simulink model "q_as_ol"  (Simulink 7.8)
settings: Solver=ode1  StartTime=0.0  StopTime=30  FixedStep=0.001  RelTol=1e-3
undefined symbols (not defined in the file): A, B, C, D, HIL, qc_get_step_size
libraries: simulink x11, quarc_library x9
settings Model: Creator=DCrymble  LastModifiedBy=pmartin  SimulationMode=external  ExtModeTrigDuration=50000  BufferReuse=off
settings SolverCC: PositivePriorityOrder=on
settings OptimizationCC: BooleanDataType=off  InlineInvariantSignals=on  OptimizeBlockIOStorage=off  BufferReuse=off  ExpressionFolding=off  LocalBlockOutputs=off  InitFltsAndDblsToZero=on
settings DebuggingCC: FcnCallInpInsideContextMsg=Use local settings  StrictBusMsg=Warning
settings SFSimCC: SimParseCustomCode=off
settings RTWCC: SystemTargetFile=quarc_windows.tlc  TemplateMakefile=quarc_default_tmf  Description=QuaRC Win32 Target  ProcessScript=quarc_windows_make_rtw_hook
settings STFCustomTargetCC: TargetPreCompLibLocation=C:\PROGRA~2\QUARC\lib\2012b\windows\release  SystemTargetFile=quarc_windows.tlc
settings GRTTargetCC: TargetPreCompLibLocation=C:\PROGRA~2\QUARC\lib\2012b\windows\release  ParMdlRefBuildCompliant=off  CompOptLevelCompliant=off  ConcurrentExecutionCompliant=off  MatFileLogging=off  ExtMode=on  ExtModeMexFile=quarc_comm

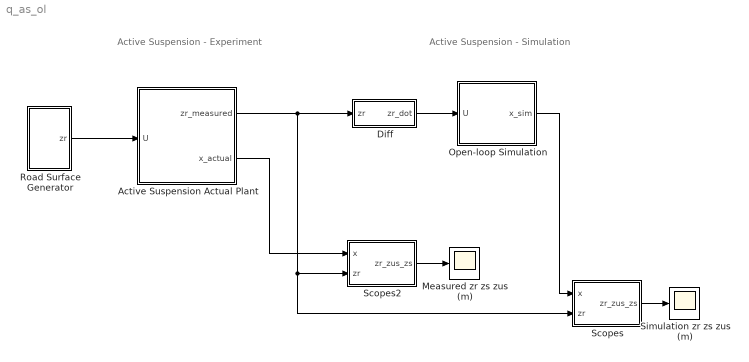
== system q_as_ol ==
  note: Active Suspension - Experiment
  note: Active Suspension - Simulation
  Active Suspension Actual Plant : Subsystem
  Diff : Subsystem
  Measured zr zs zus (m) : Scope
      settings: YMin=-0.0225  YMax=0.0325  SaveName=ScopeData3  MaxDataPoints=300000
  Open-loop Simulation : Subsystem
  Road Surface Generator : Subsystem
  Scopes : Subsystem
  Scopes2 : Subsystem
  Simulation zr zs zus (m) : Scope
      settings: YMin=-0.0225  YMax=0.0325  SaveName=ScopeData4  MaxDataPoints=300000
  wires:
  Open-loop Simulation/1(x_sim) -> Scopes/1(x)
  Active Suspension Actual Plant/1(zr_measured) -> Scopes/2(zr), Scopes2/2(zr), Diff/1(zr)
  Active Suspension Actual Plant/2(x_actual) -> Scopes2/1(x)
  Scopes2/1(zr_zus_zs) -> Measured zr zs zus (m)/1
  Scopes/1(zr_zus_zs) -> Simulation zr zs zus (m)/1
  Road Surface Generator/1(zr) -> Active Suspension Actual Plant/1(U)
  Diff/1(zr_dot) -> Open-loop Simulation/1(U)

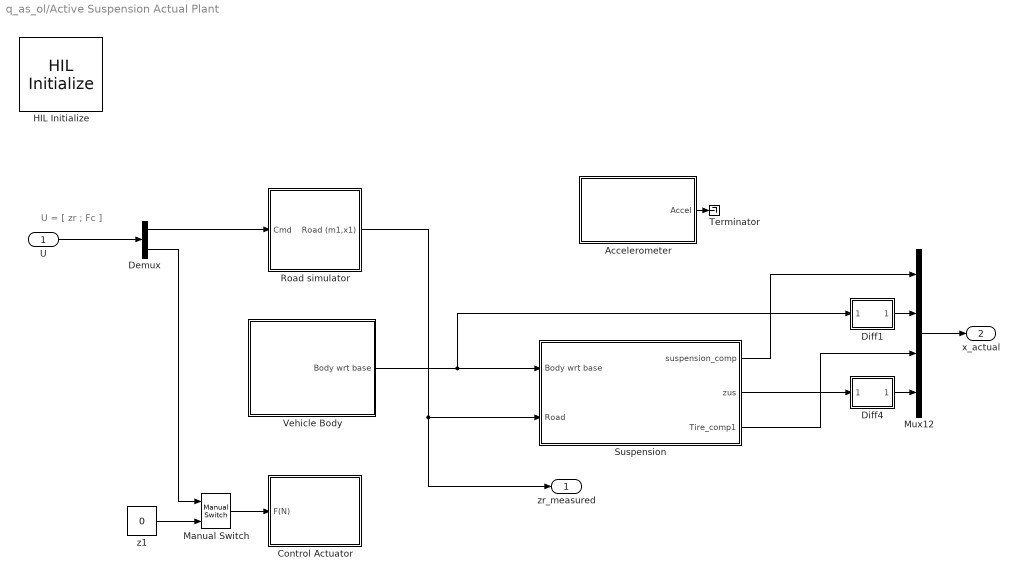
== system q_as_ol/Active Suspension Actual Plant ==
  note: U = [ zr ; Fc ]
  U : Inport
  Accelerometer : Subsystem
  Control Actuator : Subsystem
  Demux : Demux  Outputs=2
  Diff1 : Subsystem
  Diff4 : Subsystem
  HIL Initialize : quarc_library/Data Acquisition/Generic/Configuration/HIL Initialize  Priority=-99  object_name=HIL-1  board_type=q8_usb  board_number=0  board_options=update_rate=normal;decimation=1  exclusive=off  active=off  hardware_clocks=[0:2]  clock_modes=[]  initial_clock_frequencies=[]  set_clock_params_at_start=off  set_clock_params_at_switch_in=off  set_clock_frequencies_at_start=off  set_clock_frequencies_at_switch_in=off  analog_input_channels=[0:7]  analog_input_maximums=10  analog_input_minimums=-10  set_analog_input_params_at_start=on  set_analog_input_params_at_switch_in=off  analog_output_channels=[0:7]  analog_output_maximums=10  analog_output_minimums=-10  initial_analog_outputs=[0]  final_analog_outputs=[0]  watchdog_analog_outputs=0  set_analog_output_params_at_start=on  set_analog_output_params_at_switch_in=off  set_analog_outputs_at_start=on  set_analog_outputs_at_switch_in=off  set_analog_outputs_at_terminate=on  set_analog_outputs_at_switch_out=off  set_analog_outputs_on_watchdog=off  digital_input_channels=[]  digital_output_channels=[0:4]  digital_output_configuration=[]  initial_digital_outputs=[0 0 0 0 1]  final_digital_outputs=[1 1 1 1 0]  watchdog_digital_outputs=[1 1 1 1 0]  set_digital_output_params_at_start=off  set_digital_output_params_at_switch_in=off  set_digital_outputs_at_start=on  set_digital_outputs_at_switch_in=off  set_digital_outputs_at_terminate=on  set_digital_outputs_at_switch_out=off  set_digital_outputs_on_watchdog=off  encoder_channels=[0:7]  quadrature=[4]  encoder_filter_frequency=[]  initial_encoder_counts=[0]  set_encoder_params_at_start=on  set_encoder_params_at_switch_in=off  set_encoder_counts_at_start=on  set_encoder_counts_at_switch_in=off  pwm_channels=[0:7]  pwm_modes=0  pwm_frequency=99.532799999999995e6/4095  pwm_configuration=[0]  pwm_alignment=[0]  pwm_polarity=[1]  pwm_leading_deadband=[0]  pwm_trailing_deadband=[0]  initial_pwm_outputs=[0]  final_pwm_outputs=[0]  watchdog_pwm_outputs=[0]  set_pwm_params_at_start=on  set_pwm_params_at_switch_in=off  set_pwm_outputs_at_start=on  set_pwm_outputs_at_switch_in=off  set_pwm_outputs_at_terminate=on  set_pwm_outputs_at_switch_out=off  set_pwm_outputs_on_watchdog=off  other_output_channels=[]  initial_other_outputs=[]  final_other_outputs=[]  watchdog_other_outputs=[]  set_other_outputs_at_start=off  set_other_outputs_at_switch_in=off  set_other_outputs_at_terminate=off  set_other_outputs_at_switch_out=off  set_other_outputs_on_watchdog=off
  Manual Switch : simulink/Signal Routing/Manual Switch  sw=1  action=0  varsize=off
  Mux12 : Mux
  Road simulator : Subsystem
  Suspension : Subsystem
  Terminator : Terminator
  Vehicle Body : Subsystem
  z1 : Constant  Value=0
  zr_measured : Outport
  x_actual : Outport  Port=2
  wires:
  Manual Switch/1 -> Control Actuator/1(F(N))
  z1/1 -> Manual Switch/2
  Suspension/1(suspension_comp) -> Mux12/1
  Vehicle Body/1(Body wrt base) -> Diff1/1(In1), Suspension/1("Body wrt base ")
  Diff1/1(Out2) -> Mux12/2
  Diff4/1(Out2) -> Mux12/4
  Suspension/2(zus) -> Diff4/1(In1)
  Mux12/1 -> x_actual/1
  Suspension/3(Tire_comp1) -> Mux12/3
  U/1 -> Demux/1
  Road simulator/1(Road (m1,x1)) -> zr_measured/1, Suspension/2(Road)
  Accelerometer/1(Accel) -> Terminator/1
  Demux/1 -> Road simulator/1(Cmd)
  Demux/2 -> Manual Switch/1

== system q_as_ol/Diff ==
  zr : Inport
  2nd Order Filter Input ICs3 : Subsystem
  Constant : Constant  Value=0
  Constant3 : Constant  Value=1000
  Mux : Mux  Inputs=2
  Terminator_1 : Terminator
  z4 : Constant
  zr_dot : Outport
  wires:
  Constant3/1 -> 2nd Order Filter Input ICs3/2(Wn)
  z4/1 -> 2nd Order Filter Input ICs3/3(z)
  zr/1 -> 2nd Order Filter Input ICs3/1(In)
  2nd Order Filter Input ICs3/1(Out) -> Terminator_1/1
  Mux/1 -> zr_dot/1
  2nd Order Filter Input ICs3/2(Out_dot) -> Mux/1
  Constant/1 -> Mux/2

== system q_as_ol/Open-loop Simulation ==
  U : Inport
  Demux : Demux  Outputs=[4 2]
  Open-Loop  State-Space : StateSpace  A=A  B=B  C=cat(1,eye(4), C)  D=D
  Terminator : Terminator
  Unit Delay : UnitDelay  SampleTime=-1
  x_sim : Outport
  wires:
  Open-Loop  State-Space/1 -> Demux/1
  Demux/1 -> Unit Delay/1
  U/1 -> Open-Loop  State-Space/1
  Unit Delay/1 -> x_sim/1
  Demux/2 -> Terminator/1

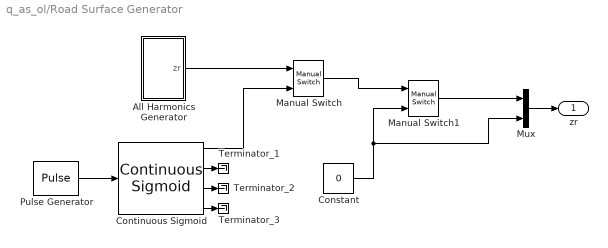
== system q_as_ol/Road Surface Generator ==
  All Harmonics Generator : Subsystem
  Constant : Constant  Value=0
  Continuous Sigmoid : quarc_library/Sources/Sigmoids/Continuous Sigmoid  params_source=Internal (dialog parameters)  max_velocity=.6/3  max_acceleration=20  initial_position=0  initial_velocity=0  hold_off=0.5  input_sample_time=-1  output_sample_time=qc_get_step_size
  Manual Switch : simulink/Signal Routing/Manual Switch  sw=1  action=0  varsize=off
  Manual Switch1 : simulink/Signal Routing/Manual Switch  sw=1  action=0  varsize=off
  Mux : Mux  Inputs=2
  Pulse Generator : DiscretePulseGenerator  PulseType=Time based  Amplitude=0.02  Period=3  PulseWidth=50  PhaseDelay=.1
  Terminator_1 : Terminator
  Terminator_2 : Terminator
  Terminator_3 : Terminator
  zr : Outport
  wires:
  Pulse Generator/1 -> Continuous Sigmoid/1
  All Harmonics Generator/1(zr) -> Manual Switch/1
  Continuous Sigmoid/1 -> Manual Switch/2
  Constant/1 -> Mux/2, Manual Switch1/2
  Manual Switch/1 -> Manual Switch1/1
  Continuous Sigmoid/2 -> Terminator_1/1
  Continuous Sigmoid/3 -> Terminator_2/1
  Continuous Sigmoid/4 -> Terminator_3/1
  Mux/1 -> zr/1
  Manual Switch1/1 -> Mux/1

== system q_as_ol/Scopes ==
  x : Inport
  zr : Inport  Port=2
  Demux : Demux
  Mux1 : Mux  Inputs=3
  Sum1 : Sum  Inputs=2  SaturateOnIntegerOverflow=on  InputSameDT=on  OutDataTypeStr=Inherit: Same as first input
  Sum3 : Sum  Inputs=3  SaturateOnIntegerOverflow=on  InputSameDT=on  OutDataTypeStr=Inherit: Same as first input
  Terminator : Terminator
  Terminator1 : Terminator
  zr_zus_zs : Outport
  wires:
  Demux/1 -> Sum3/2
  Demux/3 -> Sum3/3, Sum1/2
  zr/1 -> Mux1/1, Sum3/1, Sum1/1
  x/1 -> Demux/1
  Sum1/1 -> Mux1/2
  Sum3/1 -> Mux1/3
  Mux1/1 -> zr_zus_zs/1
  Demux/2 -> Terminator/1
  Demux/4 -> Terminator1/1

== system q_as_ol/Scopes2 ==
  x : Inport
  zr : Inport  Port=2
  Demux : Demux
  Mux1 : Mux  Inputs=3
  Sum1 : Sum  Inputs=2  SaturateOnIntegerOverflow=on  InputSameDT=on  OutDataTypeStr=Inherit: Same as first input
  Sum3 : Sum  Inputs=3  SaturateOnIntegerOverflow=on  InputSameDT=on  OutDataTypeStr=Inherit: Same as first input
  Terminator : Terminator
  Terminator1 : Terminator
  zr_zus_zs : Outport
  wires:
  Mux1/1 -> zr_zus_zs/1
  Sum3/1 -> Mux1/3
  Sum1/1 -> Mux1/2
  x/1 -> Demux/1
  zr/1 -> Sum1/1, Sum3/1, Mux1/1
  Demux/3 -> Sum1/2, Sum3/3
  Demux/1 -> Sum3/2
  Demux/2 -> Terminator/1
  Demux/4 -> Terminator1/1

== system q_as_ol/Active Suspension Actual Plant/Accelerometer ==
  Bias Removal : quarc_library/Discrete/Bias Removal  start_time=0  end_time=.099  switch_id=0  sample_time=qc_get_step_size
  HIL Read Analog : quarc_library/Data Acquisition/Generic/Immediate I//O/HIL Read Analog  object_name=HIL-1  channels=0  sample_time=qc_get_step_size  active=on  vector_output=off
  Terminator : Terminator
  Terminator1 : Terminator
  filter : Subsystem
  mm/sec1 : Gain  Gain=-9.8
  Accel : Outport
  wires:
  Bias Removal/1 -> filter/1(In1)
  filter/1(Out2) -> mm/sec1/1
  mm/sec1/1 -> Accel/1
  HIL Read Analog/1 -> Bias Removal/1
  Bias Removal/2 -> Terminator/1
  Bias Removal/3 -> Terminator1/1

== system q_as_ol/Active Suspension Actual Plant/Control Actuator ==
  F(N) : Inport
  A/V : Gain  Gain=-2
  A/V1 : Gain  Gain=1/19.16
  Amp : Scope
      settings: TimeRange=5  YMin=-1  YMax=1.25  SaveName=ScopeData9
  Force : Scope
      settings: TimeRange=5  YMin=-15  YMax=15  SaveName=ScopeData5
  HIL Write Analog1 : quarc_library/Data Acquisition/Generic/Immediate I//O/HIL Write Analog  object_name=HIL-1  channels=0  sample_time=-1  active=off  vector_input=on
  Saturation2 : Saturate  UpperLimit=5  LowerLimit=-5
  wires:
  Saturation2/1 -> Amp/1, A/V/1
  A/V1/1 -> Saturation2/1
  F(N)/1 -> Force/1, A/V1/1
  A/V/1 -> HIL Write Analog1/1

== system q_as_ol/Active Suspension Actual Plant/Diff1 ==
  In1 : Inport
  2nd Order Filter Input ICs3 : Subsystem
  Constant3 : Constant  Value=500
  Terminator_1 : Terminator
  z4 : Constant
  Out2 : Outport
  wires:
  2nd Order Filter Input ICs3/2(Out_dot) -> Out2/1
  In1/1 -> 2nd Order Filter Input ICs3/1(In)
  z4/1 -> 2nd Order Filter Input ICs3/3(z)
  Constant3/1 -> 2nd Order Filter Input ICs3/2(Wn)
  2nd Order Filter Input ICs3/1(Out) -> Terminator_1/1

== system q_as_ol/Active Suspension Actual Plant/Diff4 ==
  In1 : Inport
  2nd Order Filter Input ICs3 : Subsystem
  Constant3 : Constant  Value=500
  Terminator_1 : Terminator
  z4 : Constant
  Out2 : Outport
  wires:
  Constant3/1 -> 2nd Order Filter Input ICs3/2(Wn)
  z4/1 -> 2nd Order Filter Input ICs3/3(z)
  In1/1 -> 2nd Order Filter Input ICs3/1(In)
  2nd Order Filter Input ICs3/2(Out_dot) -> Out2/1
  2nd Order Filter Input ICs3/1(Out) -> Terminator_1/1

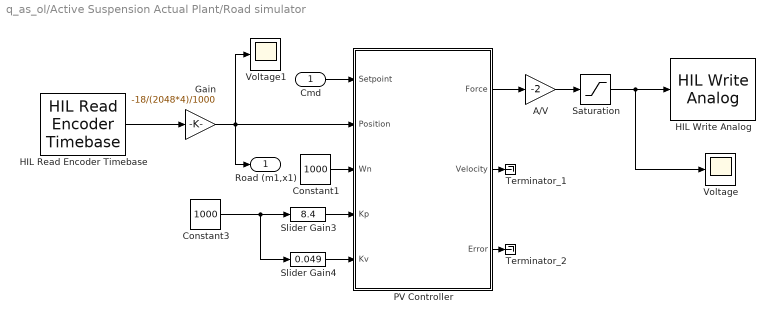
== system q_as_ol/Active Suspension Actual Plant/Road simulator ==
  Cmd : Inport
  A/V : Gain  Gain=-2
  Constant1 : Constant  Value=1000
  Constant3 : Constant  Value=1000
  Gain : Gain  Gain=-18/(2048*4)/1000
  HIL Read Encoder Timebase : quarc_library/Data Acquisition/Generic/Timebases/HIL Read Encoder Timebase  object_name=HIL-1  clock=[0]  channels=1  samples_in_buffer=max(ceil(1/qc_get_step_size), 1)  active=on  vector_output=on  data_type_mode=Inherit via back propagation  data_type=double
  HIL Write Analog : quarc_library/Data Acquisition/Generic/Immediate I//O/HIL Write Analog  object_name=HIL-1  channels=1  sample_time=-1  active=off  vector_input=on
  PV Controller : Subsystem
  Saturation : Saturate  UpperLimit=10  LowerLimit=-10
  Slider Gain3 : simulink/Math Operations/Slider Gain  low=0  gain=8.4  high=70
  Slider Gain4 : simulink/Math Operations/Slider Gain  low=0  gain=0.049  high=0.1
  Terminator_1 : Terminator
  Terminator_2 : Terminator
  Voltage : Scope
      settings: TimeRange=1  YMin=-10  YMax=-10
  Voltage1 : Scope
      settings: TimeRange=5  YMin=-0.0005  YMax=0.0105  SaveName=ScopeData16  MaxDataPoints=50000
  Road (m1,x1) : Outport
  wires:
  A/V/1 -> Saturation/1
  Constant1/1 -> PV Controller/3(Wn)
  Gain/1 -> PV Controller/2(Position), Road (m1,x1)/1, Voltage1/1
  Slider Gain3/1 -> PV Controller/4(Kp)
  Constant3/1 -> Slider Gain4/1, Slider Gain3/1
  Slider Gain4/1 -> PV Controller/5(Kv)
  HIL Read Encoder Timebase/1 -> Gain/1
  Saturation/1 -> HIL Write Analog/1, Voltage/1
  Cmd/1 -> PV Controller/1(Setpoint)
  PV Controller/1(Force) -> A/V/1
  PV Controller/2(Velocity) -> Terminator_1/1
  PV Controller/3(Error) -> Terminator_2/1

== system q_as_ol/Active Suspension Actual Plant/Suspension ==
  "Body wrt base " : Inport
  Road : Inport  Port=2
  HIL Read Encoder : quarc_library/Data Acquisition/Generic/Immediate I//O/HIL Read Encoder  object_name=HIL-1  channels=0  sample_time=qc_get_step_size  active=on  vector_output=off  data_type_mode=Inherit via back propagation  data_type=double
  Sum : Sum  Inputs=|+-
  Sum1 : Sum  Inputs=|+-
  count2m : Gain  Gain=12*pi/4000/1000
  susp_comp : Scope
      settings: YMin=-0.02  YMax=0.0125  SaveName=ScopeData11
  suspension_comp : Outport
  zus : Outport  Port=2
  Tire_comp1 : Outport  Port=3
  wires:
  Sum/1 -> zus/1, Sum1/1
  "Body wrt base "/1 -> Sum/1
  HIL Read Encoder/1 -> count2m/1
  count2m/1 -> Sum/2, suspension_comp/1, susp_comp/1
  Road/1 -> Sum1/2
  Sum1/1 -> Tire_comp1/1

== system q_as_ol/Active Suspension Actual Plant/Vehicle Body ==
  Body wrt base1 : Scope
      settings: YMin=-0.006  YMax=0.017  SaveName=ScopeData8
  HIL Read Encoder : quarc_library/Data Acquisition/Generic/Immediate I//O/HIL Read Encoder  object_name=HIL-1  channels=2  sample_time=qc_get_step_size  active=on  vector_output=off  data_type_mode=Inherit via back propagation  data_type=double
  count2m : Gain  Gain=pi()*25.4/4/4096/1000
  Body wrt base : Outport
  wires:
  HIL Read Encoder/1 -> count2m/1
  count2m/1 -> Body wrt base/1, Body wrt base1/1

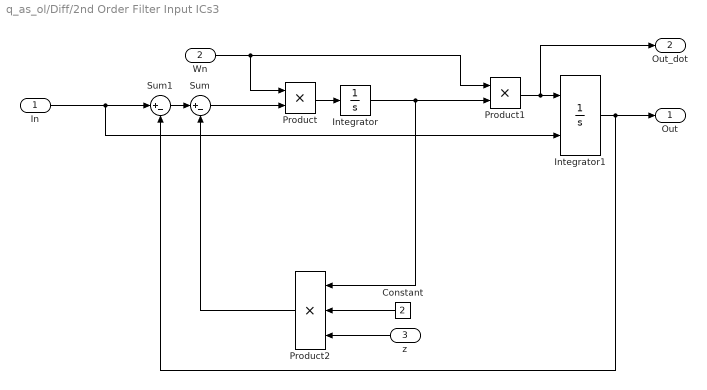
== system q_as_ol/Diff/2nd Order Filter Input ICs3 ==
  In : Inport
  Wn : Inport  Port=2
  z : Inport  Port=3
  Constant : Constant  Value=2
  Integrator : Integrator
  Integrator1 : Integrator  InitialConditionSource=external
  Product : Product  RndMeth=Zero
  Product1 : Product  RndMeth=Zero
  Product2 : Product  Inputs=3  RndMeth=Zero
  Sum : Sum  Inputs=|+-
  Sum1 : Sum  Inputs=|+-
  Out : Outport
  Out_dot : Outport  Port=2
  wires:
  Constant/1 -> Product2/2
  z/1 -> Product2/3
  Product2/1 -> Sum/2
  In/1 -> Integrator1/2, Sum1/1
  Sum1/1 -> Sum/1
  Integrator1/1 -> Out/1, Sum1/2
  Integrator/1 -> Product2/1, Product1/2
  Product1/1 -> Out_dot/1, Integrator1/1
  Wn/1 -> Product1/1, Product/1
  Sum/1 -> Product/2
  Product/1 -> Integrator/1

== system q_as_ol/Road Surface Generator/All Harmonics Generator ==
  Constant4 : Constant
  Constant5 : Constant
  Rate Transition : RateTransition
  Repeating Sequence : simulink/Sources/Repeating Sequence  rep_seq_t=[0 30 30.1 ]  rep_seq_y=[1 9.5 1 ]
  Slider Gain : simulink/Math Operations/Slider Gain  low=0  gain=0.0015  high=0.002
  Slider Gain2 : simulink/Math Operations/Slider Gain  low=-10  gain=0  high=10
  Smooth Parameterized Sin : Subsystem
      mask Type: Smooth Parameterized Sin Wave
      mask Description:
      | Sin wave that will smoothly and continuously change as input
      | parameters are changed.
      | 
      | Out = Amplitude * sin(freq*t) +offset
  Zero-Order Hold : ZeroOrderHold  SampleTime=.1
  zr : Outport
  wires:
  Slider Gain/1 -> Smooth Parameterized Sin/2(Amplitude)
  Slider Gain2/1 -> Smooth Parameterized Sin/3(Offset)
  Constant4/1 -> Slider Gain2/1
  Constant5/1 -> Slider Gain/1
  Repeating Sequence/1 -> Zero-Order Hold/1
  Zero-Order Hold/1 -> Rate Transition/1
  Rate Transition/1 -> Smooth Parameterized Sin/1(freq Hz)
  Smooth Parameterized Sin/1(Sin) -> zr/1

== system q_as_ol/Active Suspension Actual Plant/Accelerometer/filter ==
  In1 : Inport
  2nd Order Filter Input ICs3 : Subsystem
  Constant3 : Constant  Value=70
  Terminator_1 : Terminator
  z4 : Constant
  Out2 : Outport
  wires:
  In1/1 -> 2nd Order Filter Input ICs3/1(In)
  z4/1 -> 2nd Order Filter Input ICs3/3(z)
  Constant3/1 -> 2nd Order Filter Input ICs3/2(Wn)
  2nd Order Filter Input ICs3/1(Out) -> Out2/1
  2nd Order Filter Input ICs3/2(Out_dot) -> Terminator_1/1

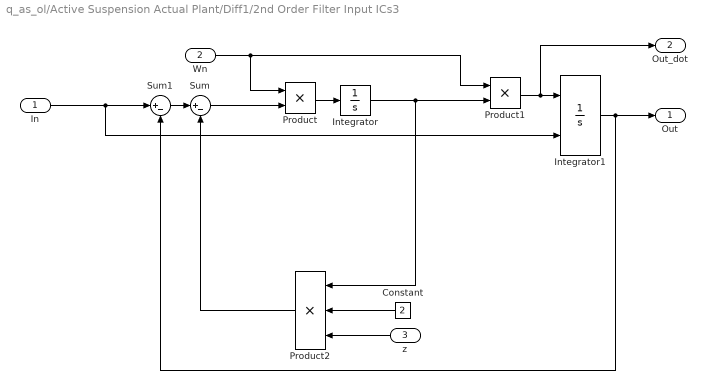
== system q_as_ol/Active Suspension Actual Plant/Diff1/2nd Order Filter Input ICs3 ==
  In : Inport
  Wn : Inport  Port=2
  z : Inport  Port=3
  Constant : Constant  Value=2
  Integrator : Integrator
  Integrator1 : Integrator  InitialConditionSource=external
  Product : Product  RndMeth=Zero
  Product1 : Product  RndMeth=Zero
  Product2 : Product  Inputs=3  RndMeth=Zero
  Sum : Sum  Inputs=|+-
  Sum1 : Sum  Inputs=|+-
  Out : Outport
  Out_dot : Outport  Port=2
  wires:
  Constant/1 -> Product2/2
  z/1 -> Product2/3
  Product2/1 -> Sum/2
  In/1 -> Integrator1/2, Sum1/1
  Sum1/1 -> Sum/1
  Integrator1/1 -> Out/1, Sum1/2
  Integrator/1 -> Product2/1, Product1/2
  Product1/1 -> Out_dot/1, Integrator1/1
  Wn/1 -> Product1/1, Product/1
  Sum/1 -> Product/2
  Product/1 -> Integrator/1

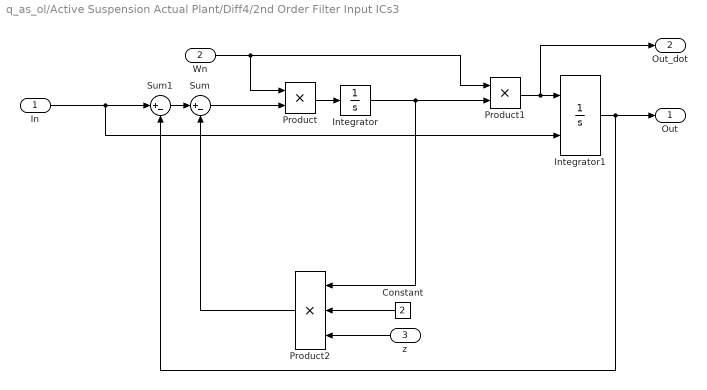
== system q_as_ol/Active Suspension Actual Plant/Diff4/2nd Order Filter Input ICs3 ==
  In : Inport
  Wn : Inport  Port=2
  z : Inport  Port=3
  Constant : Constant  Value=2
  Integrator : Integrator
  Integrator1 : Integrator  InitialConditionSource=external
  Product : Product  RndMeth=Zero
  Product1 : Product  RndMeth=Zero
  Product2 : Product  Inputs=3  RndMeth=Zero
  Sum : Sum  Inputs=|+-
  Sum1 : Sum  Inputs=|+-
  Out : Outport
  Out_dot : Outport  Port=2
  wires:
  Constant/1 -> Product2/2
  z/1 -> Product2/3
  Product2/1 -> Sum/2
  In/1 -> Integrator1/2, Sum1/1
  Sum1/1 -> Sum/1
  Integrator1/1 -> Out/1, Sum1/2
  Integrator/1 -> Product2/1, Product1/2
  Product1/1 -> Out_dot/1, Integrator1/1
  Wn/1 -> Product1/1, Product/1
  Sum/1 -> Product/2
  Product/1 -> Integrator/1

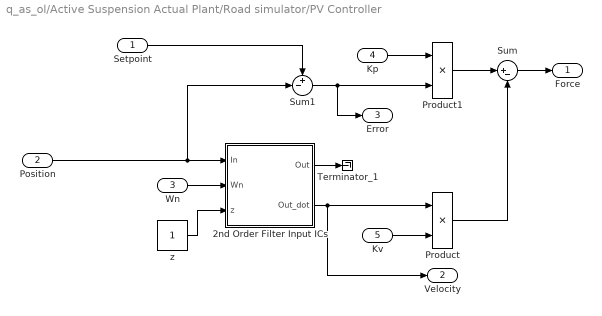
== system q_as_ol/Active Suspension Actual Plant/Road simulator/PV Controller ==
  Setpoint : Inport
  Position : Inport  Port=2
  Wn : Inport  Port=3
  Kp : Inport  Port=4
  Kv : Inport  Port=5
  2nd Order Filter Input ICs : Subsystem
  Product : Product  RndMeth=Zero
  Product1 : Product  RndMeth=Zero
  Sum : Sum  Inputs=|+-
  Sum1 : Sum  Inputs=+-|
  Terminator_1 : Terminator
  z : Constant
  Force : Outport
  Velocity : Outport  Port=2
  Error : Outport  Port=3
  wires:
  Wn/1 -> 2nd Order Filter Input ICs/2(Wn)
  z/1 -> 2nd Order Filter Input ICs/3(z)
  Position/1 -> 2nd Order Filter Input ICs/1(In), Sum1/2
  2nd Order Filter Input ICs/2(Out_dot) -> Velocity/1, Product/1
  Kp/1 -> Product1/1
  Setpoint/1 -> Sum1/1
  Sum1/1 -> Product1/2, Error/1
  Product1/1 -> Sum/1
  Kv/1 -> Product/2
  Product/1 -> Sum/2
  Sum/1 -> Force/1
  2nd Order Filter Input ICs/1(Out) -> Terminator_1/1

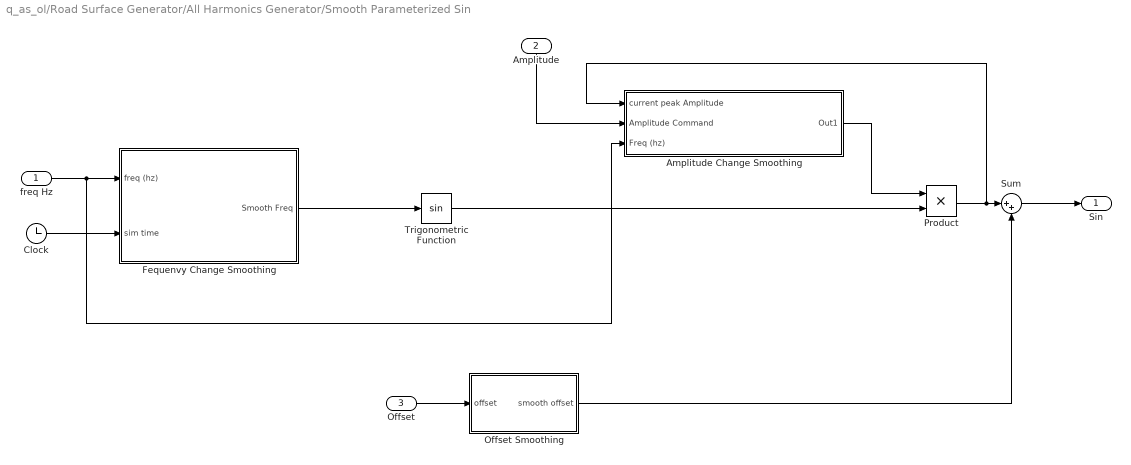
== system q_as_ol/Road Surface Generator/All Harmonics Generator/Smooth Parameterized Sin ==
  freq Hz : Inport
  Amplitude : Inport  Port=2
  Offset : Inport  Port=3
  Amplitude Change Smoothing : Subsystem
  Clock : Clock
  Fequenvy Change Smoothing : Subsystem
  Offset Smoothing : Subsystem
  Product : Product  RndMeth=Zero
  Sum : Sum  Inputs=|++
  Trigonometric Function : Trigonometry
  Sin : Outport
  wires:
  Sum/1 -> Sin/1
  Clock/1 -> Fequenvy Change Smoothing/2(sim time)
  freq Hz/1 -> Fequenvy Change Smoothing/1(freq (hz)), Amplitude Change Smoothing/3(Freq (hz))
  Fequenvy Change Smoothing/1(Smooth Freq) -> Trigonometric Function/1
  Trigonometric Function/1 -> Product/2
  Offset Smoothing/1(smooth offset) -> Sum/2
  Offset/1 -> Offset Smoothing/1(offset)
  Product/1 -> Sum/1, Amplitude Change Smoothing/1(current peak Amplitude)
  Amplitude Change Smoothing/1(Out1) -> Product/1
  Amplitude/1 -> Amplitude Change Smoothing/2(Amplitude Command)

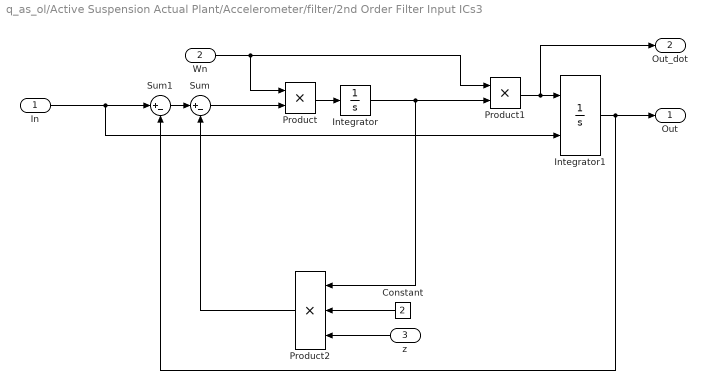
== system q_as_ol/Active Suspension Actual Plant/Accelerometer/filter/2nd Order Filter Input ICs3 ==
  In : Inport
  Wn : Inport  Port=2
  z : Inport  Port=3
  Constant : Constant  Value=2
  Integrator : Integrator
  Integrator1 : Integrator  InitialConditionSource=external
  Product : Product  RndMeth=Zero
  Product1 : Product  RndMeth=Zero
  Product2 : Product  Inputs=3  RndMeth=Zero
  Sum : Sum  Inputs=|+-
  Sum1 : Sum  Inputs=|+-
  Out : Outport
  Out_dot : Outport  Port=2
  wires:
  Constant/1 -> Product2/2
  z/1 -> Product2/3
  Product2/1 -> Sum/2
  In/1 -> Integrator1/2, Sum1/1
  Sum1/1 -> Sum/1
  Integrator1/1 -> Out/1, Sum1/2
  Integrator/1 -> Product2/1, Product1/2
  Product1/1 -> Out_dot/1, Integrator1/1
  Wn/1 -> Product1/1, Product/1
  Sum/1 -> Product/2
  Product/1 -> Integrator/1

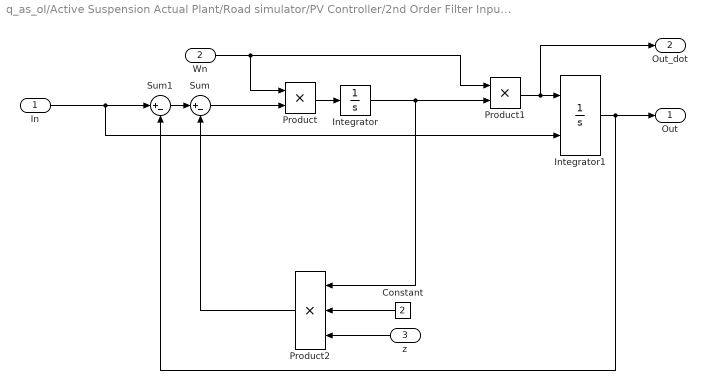
== system q_as_ol/Active Suspension Actual Plant/Road simulator/PV Controller/2nd Order Filter Input ICs ==
  In : Inport
  Wn : Inport  Port=2
  z : Inport  Port=3
  Constant : Constant  Value=2
  Integrator : Integrator
  Integrator1 : Integrator  InitialConditionSource=external
  Product : Product  RndMeth=Zero
  Product1 : Product  RndMeth=Zero
  Product2 : Product  Inputs=3  RndMeth=Zero
  Sum : Sum  Inputs=|+-
  Sum1 : Sum  Inputs=|+-
  Out : Outport
  Out_dot : Outport  Port=2
  wires:
  Constant/1 -> Product2/2
  z/1 -> Product2/3
  Product2/1 -> Sum/2
  In/1 -> Integrator1/2, Sum1/1
  Sum1/1 -> Sum/1
  Integrator1/1 -> Out/1, Sum1/2
  Integrator/1 -> Product2/1, Product1/2
  Product1/1 -> Out_dot/1, Integrator1/1
  Wn/1 -> Product1/1, Product/1
  Sum/1 -> Product/2
  Product/1 -> Integrator/1

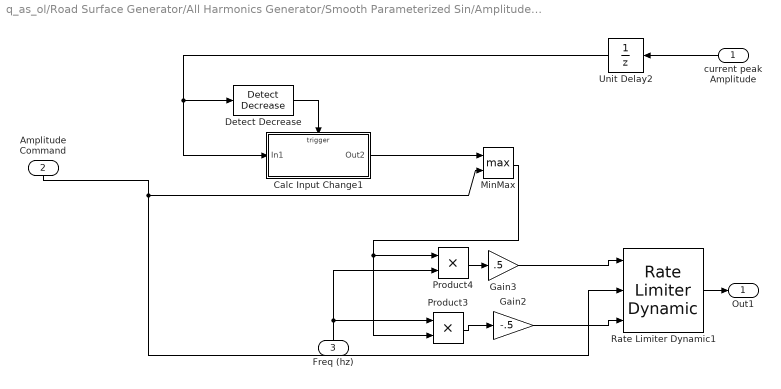
== system q_as_ol/Road Surface Generator/All Harmonics Generator/Smooth Parameterized Sin/Amplitude Change Smoothing ==
  current peak Amplitude : Inport
  Amplitude Command : Inport  Port=2
  Freq (hz) : Inport  Port=3
  Calc Input Change1 : Subsystem  TreatAsAtomicUnit=on
  Detect Decrease : simulink/Logic and Bit Operations/Detect Decrease  vinit=0.0  InputProcessing=Inherited  OutDataTypeStr=uint8
  Gain2 : Gain  Gain=-.5
  Gain3 : Gain  Gain=.5
  MinMax : MinMax  Function=max  Inputs=2
  Product3 : Product  RndMeth=Zero
  Product4 : Product  RndMeth=Zero
  Rate Limiter Dynamic1 : simulink/Discontinuities/Rate Limiter Dynamic
  Unit Delay2 : UnitDelay  SampleTime=-1
  Out1 : Outport
  wires:
  Gain2/1 -> Rate Limiter Dynamic1/3
  Gain3/1 -> Rate Limiter Dynamic1/1
  Amplitude Command/1 -> MinMax/2, Rate Limiter Dynamic1/2
  Product3/1 -> Gain2/1
  Product4/1 -> Gain3/1
  Detect Decrease/1 -> Calc Input Change1/Trigger
  Calc Input Change1/1(Out2) -> MinMax/1
  Unit Delay2/1 -> Calc Input Change1/1(In1), Detect Decrease/1
  MinMax/1 -> Product4/1, Product3/2
  current peak Amplitude/1 -> Unit Delay2/1
  Freq (hz)/1 -> Product3/1, Product4/2
  Rate Limiter Dynamic1/1 -> Out1/1

== system q_as_ol/Road Surface Generator/All Harmonics Generator/Smooth Parameterized Sin/Fequenvy Change Smoothing ==
  freq (hz) : Inport
  sim time : Inport  Port=2
  Hz2rad/s : Gain  Gain=2*pi
  Product1 : Product  RndMeth=Zero
  Relational Operator : RelationalOperator  Operator=~=  OutDataTypeStr=boolean
  Sum1 : Sum  Inputs=|+-
  Sum2 : Sum  Inputs=-+|
  Triggered Subsystem : Subsystem  TreatAsAtomicUnit=on
  Unit Delay : UnitDelay  SampleTime=-1
  Unit Delay1 : UnitDelay  SampleTime=-1
  Smooth Freq : Outport
  wires:
  Triggered Subsystem/1(Out2) -> Sum2/1
  Unit Delay1/1 -> Sum1/2
  Relational Operator/1 -> Triggered Subsystem/Trigger
  Sum1/1 -> Triggered Subsystem/1(In1)
  Unit Delay/1 -> Relational Operator/1
  Product1/1 -> Sum2/2, Sum1/1, Unit Delay1/1
  freq (hz)/1 -> Unit Delay/1, Relational Operator/2, Hz2rad/s/1
  Sum2/1 -> Smooth Freq/1
  sim time/1 -> Product1/2
  Hz2rad/s/1 -> Product1/1

== system q_as_ol/Road Surface Generator/All Harmonics Generator/Smooth Parameterized Sin/Offset Smoothing ==
  offset : Inport
  Abs : Abs
  Abs1 : Abs
  Gain : Gain
  Gain1 : Gain  Gain=-1
  MinMax1 : MinMax  Function=max  Inputs=2
  Rate Limiter Dynamic : simulink/Discontinuities/Rate Limiter Dynamic
  Unit Delay3 : UnitDelay  SampleTime=-1
  smooth offset : Outport
  wires:
  Rate Limiter Dynamic/1 -> Abs1/1, smooth offset/1
  offset/1 -> Rate Limiter Dynamic/2, Abs/1
  Gain1/1 -> Rate Limiter Dynamic/3
  Gain/1 -> Rate Limiter Dynamic/1
  MinMax1/1 -> Unit Delay3/1
  Unit Delay3/1 -> Gain/1, Gain1/1
  Abs/1 -> MinMax1/2
  Abs1/1 -> MinMax1/1

== system q_as_ol/Road Surface Generator/All Harmonics Generator/Smooth Parameterized Sin/Amplitude Change Smoothing/Calc Input Change1 ==
  In1 : Inport
  Trigger : TriggerPort
  Out2 : Outport  InitialOutput=1000
  wires:
  In1/1 -> Out2/1

== system q_as_ol/Road Surface Generator/All Harmonics Generator/Smooth Parameterized Sin/Fequenvy Change Smoothing/Triggered Subsystem ==
  In1 : Inport
  Trigger : TriggerPort
  Sum1 : Sum
  Unit Delay1 : UnitDelay  SampleTime=-1
  Out2 : Outport  InitialOutput=0
  wires:
  Unit Delay1/1 -> Sum1/1
  Sum1/1 -> Unit Delay1/1, Out2/1
  In1/1 -> Sum1/2
